simulink model "Test3C120Board_QuadDisplay"  (Simulink 6.4)
settings: Solver=ode45  SolverMode=SingleTasking  StartTime=0.0  StopTime=100.0  FixedStep=1  RelTol=1e-3
InitFcn:
  | %% DSPBuilder Start
  | alt_dspbuilder_update_model(bdroot)
  | %% DSPBuilder End
undefined symbols (not defined in the file): Pin_A3, Pin_AB15, Pin_AC14, Pin_AC19, Pin_AD14, Pin_AD18, Pin_AD4, Pin_AD5, Pin_AE6, Pin_AF25, Pin_AG23, Pin_B3, Pin_C3, Pin_C4, Pin_C5, Pin_D4, Pin_D5, Pin_E4, Pin_E5, Pin_G19, Pin_G20
libraries: allblocks_alteradspbuilder2 x17, Cyclone_III_EP3C120_alteradspbuilder2 x5
settings Model: Creator=lkong  LastModifiedBy=lkong
settings DataIOCC: SignalLoggingName=sigsOut
settings OptimizationCC: InlineInvariantSignals=on
settings DebuggingCC: SolverPrmCheckMsg=none  StrictBusMsg=None
settings HardwareCC: TargetUnknown=on
settings GRTTargetCC: ModelReferenceCompliant=off  MatFileLogging=off

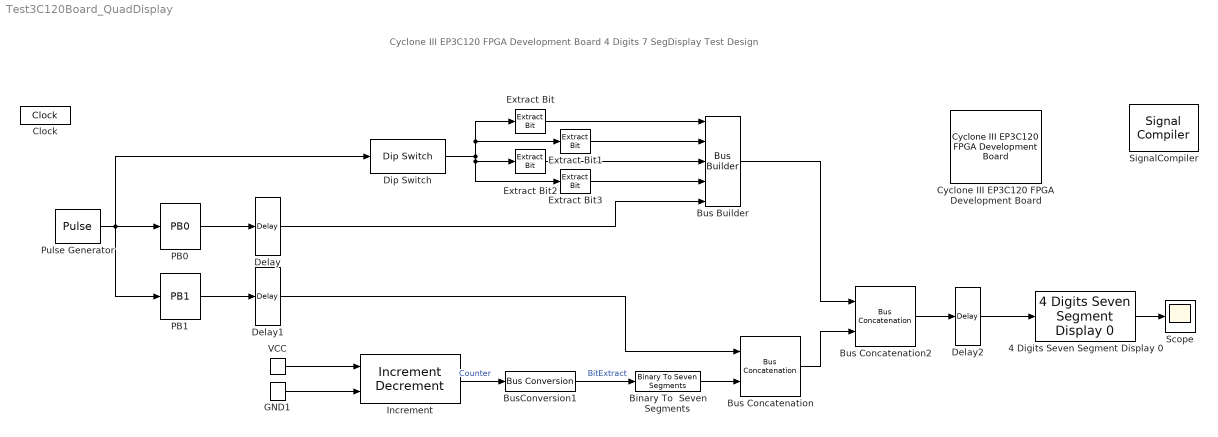
== system Test3C120Board_QuadDisplay ==
  note: Cyclone III EP3C120 FPGA Development Board 4 Digits 7 SegDisplay Test Design
  4 Digits Seven Segment Display 0 : Cyclone_III_EP3C120_alteradspbuilder2/4 Digits Seven Segment Display 0  iofile=d:\ws80\workspace\Documentation\DesignExamples\Demos\Board\CycloneIII_DSPBoard_3C120\tb_Test3C120Board_QuadDisplay\Test3C120Board%5FQuadDisplay_4+Digits+Seven+Segment+Display+0.capture  externalType=Inferred  location=Pin_AD5,Pin_A3,Pin_C4,Pin_D4,Pin_E5,Pin_D5,Pin_AE6,Pin_AD4,Pin_B3,Pin_C5,Pin_E4,Pin_C3,Pin_G19
  Binary To  Seven Segments : allblocks_alteradspbuilder2/Binary To Seven Segments  pipeline_display=0
  Bus Builder : allblocks_alteradspbuilder2/Bus Builder  BusType=Unsigned Integer  bwl=5  bwr=1  pipeline_display=0
  Bus Concatenation : allblocks_alteradspbuilder2/Bus Concatenation  isSigned=off  awidth=1  bwidth=7  pipeline_display=0
  Bus Concatenation2 : allblocks_alteradspbuilder2/Bus Concatenation  isSigned=off  awidth=5  bwidth=8  pipeline_display=0
  BusConversion1 : allblocks_alteradspbuilder2/Bus Conversion  BusType=Unsigned Integer  ibwl=29  ibwr=0  bwl=4  bwr=0  bitToConnectToOutputLSB=25  round=off  saturate=off  pipeline_display=0
  Clock : allblocks_alteradspbuilder2/Clock  ClockPeriod=10  ClockPeriodUnit=ns  SampleTime=1  SimulationStartCycle=5  PhaseOffset=0  Reset=aclr  ResetType=Active Low  Export=off
  Cyclone III EP3C120 FPGA Development Board : Cyclone_III_EP3C120_alteradspbuilder2/Cyclone III EP3C120 FPGA Development Board  ClockPinIn=Pin_AH15  GlobalResetPin=Pin_T21  device=EP3C120F780C7
  Delay : allblocks_alteradspbuilder2/Delay  pipeline=1  pipeline_display=1  ClockPhase=1  use_ena=off  use_sclr=off  allowFloatingPointOverride=on  logOutputs=off  logFile=d:\ws80\workspace\Documentation\DesignExamples\Demos\Board\CycloneIII_DSPBoard_3C120\tb_Test3C120Board_QuadDisplay\Test3C120Board%5FQuadDisplay_Delay.fixedpointlog  use_init=off  reset_value=1
  Delay1 : allblocks_alteradspbuilder2/Delay  pipeline=1  pipeline_display=1  ClockPhase=1  use_ena=off  use_sclr=off  allowFloatingPointOverride=on  logOutputs=off  logFile=d:\ws80\workspace\Documentation\DesignExamples\Demos\Board\CycloneIII_DSPBoard_3C120\tb_Test3C120Board_QuadDisplay\Test3C120Board%5FQuadDisplay_Delay1.fixedpointlog  use_init=off  reset_value=1
  Delay2 : allblocks_alteradspbuilder2/Delay  pipeline=1  pipeline_display=1  ClockPhase=1  use_ena=off  use_sclr=off  allowFloatingPointOverride=on  logOutputs=off  logFile=d:\ws80\workspace\Documentation\DesignExamples\Demos\Board\CycloneIII_DSPBoard_3C120\tb_Test3C120Board_QuadDisplay\Test3C120Board%5FQuadDisplay_Delay2.fixedpointlog  use_init=off  reset_value=1
  Dip Switch : Cyclone_III_EP3C120_alteradspbuilder2/Dip Switch  iofile=d:\ws80\workspace\Documentation\DesignExamples\Demos\Board\CycloneIII_DSPBoard_3C120\tb_Test3C120Board_QuadDisplay\Test3C120Board%5FQuadDisplay_Dip+Switch.salt  externalType=Inferred  SpecifyClock=off  location=Pin_AC14,Pin_AD18,Pin_AG23,Pin_AC19,Pin_AD14,Pin_G20,Pin_AB15,Pin_AF25
  Extract Bit : allblocks_alteradspbuilder2/Extract Bit  BusType=Unsigned Integer  bwl=7  bwr=0  bitToSelect=0  pipeline_display=0
  Extract Bit1 : allblocks_alteradspbuilder2/Extract Bit  BusType=Unsigned Integer  bwl=7  bwr=0  bitToSelect=1  pipeline_display=0
  Extract Bit2 : allblocks_alteradspbuilder2/Extract Bit  BusType=Unsigned Integer  bwl=7  bwr=0  bitToSelect=2  pipeline_display=0
  Extract Bit3 : allblocks_alteradspbuilder2/Extract Bit  BusType=Unsigned Integer  bwl=7  bwr=0  bitToSelect=3  pipeline_display=0
  GND1 : allblocks_alteradspbuilder2/GND  SpecifyClock=off
  Increment : allblocks_alteradspbuilder2/Increment Decrement  BusType=Unsigned Integer  bwl=29  bwr=0  SpecifyClock=off  clr_value=0  direction=Increment  phase_selection=1  use_ena=on  use_sclr=on  pipeline_display=1
  PB0 : Cyclone_III_EP3C120_alteradspbuilder2/PB0  iofile=d:\ws80\workspace\Documentation\DesignExamples\Demos\Board\CycloneIII_DSPBoard_3C120\tb_Test3C120Board_QuadDisplay\Test3C120Board%5FQuadDisplay_PB0.salt  externalType=Inferred  SpecifyClock=off  location=Pin_AD7
  PB1 : Cyclone_III_EP3C120_alteradspbuilder2/PB1  iofile=d:\ws80\workspace\Documentation\DesignExamples\Demos\Board\CycloneIII_DSPBoard_3C120\tb_Test3C120Board_QuadDisplay\Test3C120Board%5FQuadDisplay_PB1.salt  externalType=Inferred  SpecifyClock=off  location=Pin_AC12
  Pulse Generator : DiscretePulseGenerator  Period=20000  PulseWidth=2
  Scope : Scope
  SignalCompiler : allblocks_alteradspbuilder2/Signal Compiler  DeviceFamily=Cyclone III  DeviceName=EP3C120F780C7  EnableSignalTap=on  SignalTapDepth=512  UseBoardBlock=on  StpUseDefaultClock=on  StpClock=Clock  ExportDir=D:\MATLAB\R2006a\work
  VCC : allblocks_alteradspbuilder2/VCC  SpecifyClock=off
  wires:
  Pulse Generator/1 -> PB0/1, PB1/1, Dip Switch/1
  GND1/1 -> Increment/2
  VCC/1 -> Increment/1
  Increment/1 -> BusConversion1/1  "Counter"
  BusConversion1/1 -> Binary To  Seven Segments/1  "BitExtract"
  PB0/1 -> Delay/1
  PB1/1 -> Delay1/1
  Bus Concatenation2/1 -> Delay2/1
  Binary To  Seven Segments/1 -> Bus Concatenation/2
  Bus Builder/1 -> Bus Concatenation2/1
  Bus Concatenation/1 -> Bus Concatenation2/2
  Delay/1 -> Bus Builder/5
  Delay1/1 -> Bus Concatenation/1
  Extract Bit/1 -> Bus Builder/1
  Dip Switch/1 -> Extract Bit/1, Extract Bit1/1, Extract Bit2/1, Extract Bit3/1
  Extract Bit1/1 -> Bus Builder/2
  Extract Bit2/1 -> Bus Builder/3
  Extract Bit3/1 -> Bus Builder/4
  Delay2/1 -> 4 Digits Seven Segment Display 0/1
  4 Digits Seven Segment Display 0/1 -> Scope/1
